simulink model "iexexc_m"  (Simulink 7.9)
settings: Solver=ode45  SolverMode=SingleTasking  StartTime=0.0  StopTime=999999  MaxStep=10  RelTol=1e-3  AbsTol=1e-3
values from neighbouring files (symbols this model uses):
  U = st_Varia('LongNames')    [iexexc_i.m]
  x0 = [0.00000000000001*ones(P.NumCel,1); q0*ones(P.NumCel,1)]    [iexexc_i.m]    (also in iexexc_s.m = x0)
undefined symbols (not defined in the file or in its folder): B
settings Model: Creator=psross  LastModifiedBy=M.Sparnaaij
settings DataIOCC: LimitDataPoints=off  SaveOutput=off  SaveTime=off  SignalLoggingName=sigsOut
settings OptimizationCC: BooleanDataType=off  InitFltsAndDblsToZero=on
settings DebuggingCC: SaveWithParameterizedLinksMsg=none  SignalResolutionControl=TryResolveAllWithWarning  SolverPrmCheckMsg=none  MultiTaskDSMMsg=warning  MultiTaskCondExecSysMsg=none  FcnCallInpInsideContextMsg=Use local settings  StrictBusMsg=None
settings HardwareCC: TargetUnknown=on
settings RTWCC: IncludeERTFirstTime=on
settings GRTTargetCC: CombineOutputUpdateFcns=off  GRTInterface=on

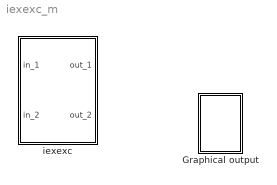
== system iexexc_m ==
  Graphical output : Subsystem
      settings: OpenFcn=iexexc_g
      mask Display:
      | plot(0,0,100,100,[80,20,20],[20,20,80],[80,69,60,52,45,39,33,28,24,20],[65,65,64,61,57,52,45,37,30,20])
      | disp('');
      | text(100,100,'iexexc', 'horizontalAlignment', 'right', 'verticalAlignment', 'top');
  iexexc : Subsystem  Description="This model calculates the removal of DOC with an activated carbon filter. Make sure the length of a filterrun is bigger than the simulation stop time entered in \"Parameters...\" on the \"Simulation\" menu."
      mask init:
      | filenaam='.\StimelaData\Activated_carbon_filter.mat';
      | 
      | [Pn,Fn,Fext]=Fileprop(filenaam);
      | 
      | errstr = st_UniqName(filenaam,'filenaam=''','SubSystem','OpenFcn');
      | if errstr, error([errstr 'The filename "' filenaam '" is already in use. Choose a different filename.']), end
      | 
      | P = iexexc_p(filenaam);
      | [B,x0,U]=iexexc_i(filenaam);
      settings: OpenFcn=|
      | filenaam='.\StimelaData\Activated_carbon_filter.mat';
      | st_ParameterInput('init',gcb,filenaam,'iexexc');
      mask Display:
      | plot(0,0,100,100,[25.000000,25.000000,75.000000,75.000000,87.500000],[75.000000,25.000000,25.000000,30.000000,30.000000],[87.500000,75.000000,75.000000],[37.500000,37.500000,75.000000],[25.000000,75.000000],[65.000000,65.000000],[25.000000,75.000000],[42.500000,42.500000],[37.500000,42.500000],[52.500000,52.500000],[50.000000,55.000000],[52.500000,52.500000],[62.500000,67.500000],[52.500000,52.500000])
      | disp('')
      | text(50,50,'iexexc', 'horizontalAlignment', 'center', 'verticalAlignment', 'middle');
      | text(50,0,Fn, 'horizontalAlignment', 'center', 'verticalAlignment', 'base');

== system iexexc_m/Graphical output ==
  note: plotten

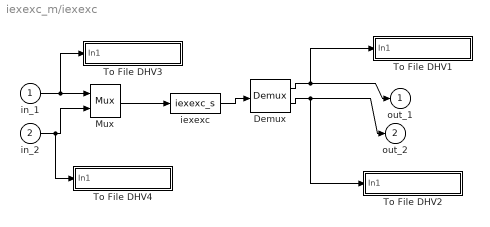
== system iexexc_m/iexexc ==
  in_1 : Inport
  in_2 : Inport  Port=2
  Demux : Demux  Outputs=[U.Number B.Measurements]
  Mux : Mux  Inputs=[U.Number B.Setpoints]
  To File DHV1 : Subsystem  mask(To File DHV){naam=[filenaam(1:length(filenaam)-4) '_out.sti']}
      mask prompts: naam "Naam van bestand"
      mask init:
      | set_param([gcb '/To File'],'Filename',naam);
      mask Display: disp(naam)
  To File DHV2 : Subsystem  mask(To File DHV){naam=[filenaam(1:length(filenaam)-4) '_EM.sti']}
      mask prompts: naam "Naam van bestand"
      mask init:
      | set_param([gcb '/To File'],'Filename',naam);
      mask Display: disp(naam)
  To File DHV3 : Subsystem  mask(To File DHV){naam=[filenaam(1:length(filenaam)-4) '_in.sti']}
      mask prompts: naam "Naam van bestand"
      mask init:
      | set_param([gcb '/To File'],'Filename',naam);
      mask Display: disp(naam)
  To File DHV4 : Subsystem  mask(To File DHV){naam=[filenaam(1:length(filenaam)-4) '_ES.sti']}
      mask prompts: naam "Naam van bestand"
      mask init:
      | set_param([gcb '/To File'],'Filename',naam);
      mask Display: disp(naam)
  iexexc : S-Function  FunctionName=iexexc_s  Parameters=B,x0,U,P  EnableBusSupport=off
  out_1 : Outport  InitialOutput=0
  out_2 : Outport  Port=2  InitialOutput=0
  wires:
  in_2/1 -> To File DHV4/1(In1), Mux/2
  Mux/1 -> iexexc/1
  in_1/1 -> To File DHV3/1(In1), Mux/1
  iexexc/1 -> Demux/1
  Demux/1 -> To File DHV1/1(In1), out_1/1
  Demux/2 -> To File DHV2/1(In1), out_2/1

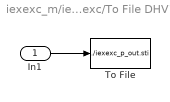
== system iexexc_m/iexexc/To File DHV1 ==
  In1 : Inport
  To File : ToFile  Filename=./iexexc_p_out.sti  MatrixName=iexexcout
  wires:
  In1/1 -> To File/1

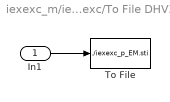
== system iexexc_m/iexexc/To File DHV2 ==
  In1 : Inport
  To File : ToFile  Filename=./iexexc_p_EM.sti  MatrixName=iexexcEM
  wires:
  In1/1 -> To File/1

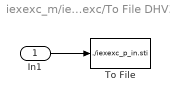
== system iexexc_m/iexexc/To File DHV3 ==
  In1 : Inport
  To File : ToFile  Filename=./iexexc_p_in.sti  MatrixName=iexexcin
  wires:
  In1/1 -> To File/1

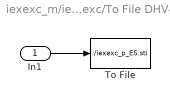
== system iexexc_m/iexexc/To File DHV4 ==
  In1 : Inport
  To File : ToFile  Filename=./iexexc_p_ES.sti  MatrixName=iexexcES
  wires:
  In1/1 -> To File/1
